simulink model "pp"  (R2021a)
settings: Solver=VariableStepAuto  StartTime=0.0  StopTime=10  RelTol=1e-3
values from neighbouring files (symbols this model uses):
  bound = 1e-6    (= 1e-06)    [parameter_setting.m]
  degree = 0.5    [parameter_setting.m]
  N = 2    [ICL_offline.m]
  rp = [-0.1 0 0.1]    [parameter_setting.m]
undefined symbols (not defined in the file or in its folder): DiscIntNeverNeededParam, Levenberg, Marquardt, sigbuilder_block, X, Y, Z
libraries: sm_lib x161, nesl_utility x35, robotmaniplib x2
(part 5 of 5)

== matlab function pp/Controller ==
  settings: updateMethod=DISCRETE  sampleTime=0.0001
  data: ref input; tau_1 output; tau_2 output; rp input; state input; wrench input; t input; aa output; b output; c output; dbg output; dbg1 output; dbg2 output; dbg3 output; dbg4 output
function [tau_1,tau_2,aa, b, c, dbg, dbg1, dbg2, dbg3, dbg4] = fcn(ref, rp, state, wrench, t)
%% gains
% robot number
N = 2;

% ICL gain
N_o = 10;
eason_integral = 4;
ICL_switcher = true;
k_cl_m = 2;
k_cl_rp = 1;
k_cl_I = 1;
k_cl_Ixx = 100; %100
k_cl_Iyy = 25; %25
k_cl_Izz = 15;
k_cl_ri = 10;
k_cl = [k_cl_m k_cl_rp*ones(1,3) k_cl_Ixx k_cl_I k_cl_I k_cl_Iyy k_cl_I k_cl_Izz k_cl_ri*ones(1,3*N)];
k_cl_gain = diag(k_cl);

% gamma o
g_m = 1;
g_rp = 1;
g_I = 1;
g_Ixx = 1;
g_Iyy = 1;
g_Izz = 1;
g_ri = 1;
gg = [g_m g_rp*ones(1,3) g_Ixx g_I g_I g_Iyy g_I g_Izz g_ri*ones(1,3*N)];
g_o = diag(gg);

% Kd matrix
Kdl = 1;
kdz = 20;
Kdr = 5;
Kdd = [Kdl*ones(1,2) kdz Kdr*ones(1,3)];
Kd = diag(Kdd);

% sliding parameter
lambda = 3;

% deadband in which to stop adaptation
deadband = 0.00;

%% function definition
function output = vee(matrix)
    output = [matrix(3, 2); matrix(1, 3); matrix(2, 1)];
end

function output = Pa(matrix)
    output = 0.5 * (matrix - matrix.');
end

function output = skew(v)
   output =  [    0 -v(3)   v(2)
               v(3)     0  -v(1)
              -v(2)  v(1)      0];
end

function output = L(v)
    output = [v(1)  v(2)  v(3)     0     0     0
                 0  v(1)     0  v(2)  v(3)     0
                 0     0  v(1)     0  v(2)  v(3)];
end
%% initialize
persistent v_last;
persistent w_last;
persistent index;
persistent mat_matrix;
persistent theta_o_hat;
persistent theta_o;
persistent Rd;
persistent xd;
persistent ICL_update;
persistent t_last;
persistent eason_ptr;

if isempty(index)
        % ground truth
        mass = 2;
        center_of_mass = rp;
        inertia_matrix = [0.0133333, 0, 0, 0.113333, 0, 0.113333];
        r1 = [-0.4 0 0] - rp;
        r2 = [0.4 0 0] - rp;
        r = [r1, r2];
        if N == 1
            theta_o = [mass mass*center_of_mass inertia_matrix r1].';
        else
            theta_o = [mass mass*center_of_mass inertia_matrix r].';
        end
        
        % initial guess
        theta_o_hat = zeros(10 + 3 * N, 1);
        theta_o_hat = theta_o;
        % mass
        theta_o_hat(1) = 0;
        % COG
        theta_o_hat(2) = 0;
        theta_o_hat(3) = 0;
        theta_o_hat(4) = 0;
        % Inertia
        theta_o_hat(5) = 0.0;
        theta_o_hat(6) = 0.0;
        theta_o_hat(7) = 0.0;
        theta_o_hat(8) = 0.0;
        theta_o_hat(9) = 0.0;
        theta_o_hat(10) = 0.0;
        % 1st grasp point
        theta_o_hat(11) = 0;
        theta_o_hat(12) = 0;
        theta_o_hat(13) = 0;
        % 2nd grasp point
        if N == 2
            theta_o_hat(14) = 0;
            theta_o_hat(15) = 0;
            theta_o_hat(16) = 0;
        end
        
        % without ICL first time
        ICL_update = false;

        Rd = [1  0  0;
              0  1  0;
              0  0  1];

        xd = [0.8750; 0.1092; 0.42] + rp.';
        index = 1;
        v_last = zeros(3, 1);
        w_last = zeros(3, eason_integral);
        mat_matrix = zeros(size(theta_o_hat, 1), N_o);
        t_last = 0;
        eason_ptr = 1; 
end

mat_sum = zeros(size(theta_o_hat, 1), 1);
debug_msg = zeros(6, 1);
dt = t - t_last;
G = [0; 0; -9.80665];

%% unpack ref
vd = [ref(1); ref(2); ref(3)];
ad = [ref(4); ref(5); ref(6)];
wd = [ref(7); ref(8); ref(9)];
ald = [ref(10); ref(11); ref(12)];

%% unpack state
quat = [state(1) state(2) state(3) state(4)];
R = quat2rotm(quat);
w = [state(5); state(6); state(7)];
x = [state(8); state(9); state(10)];
v = [state(11); state(12); state(13)];
a = [state(14); state(15); state(16)];

wrench_rotation = [         R, zeros(3,3);
                   zeros(3,3),          R];
wrench1_b = [wrench(1); wrench(2); wrench(3); wrench(4); wrench(5); wrench(6)];
wrench_1 = wrench_rotation * wrench1_b;
force_1 = [wrench_1(1); wrench_1(2); wrench_1(3)];
if N == 2
    wrench2_b = [wrench(7); wrench(8); wrench(9); wrench(10); wrench(11); wrench(12)];
    wrench_2 = wrench_rotation * wrench2_b;
    force_2 = [wrench_2(1); wrench_2(2); wrench_2(3)];
end

%% compute error signals
Re = Rd.' * R;
we = w - wd;

%% compute composite error s
sigma = we + lambda * Rd * vee(Pa(Re));
v_t = v - vd;
x_t = x - xd;
s = [v_t + lambda * x_t;
                  sigma];

%% regression matrix
alpha_r = ald - lambda * skew(wd) * Rd * vee(Pa(Re)) - lambda * Rd * vee(Pa(skew(Rd.' * we) * Re));
w_r = wd - lambda * Rd * vee(Pa(Re));
a_r = ad - lambda * v_t;
v_r = vd - lambda * x_t;

Y_l = [a_r, -skew(alpha_r) * R - skew(w) * skew(w_r) * R, zeros(3,6+3*N)];
if N == 1
    Y_r = [zeros(3,1), skew(a_r) * R + skew(w) * skew(v_r) * R - skew(w_r) * skew(v) * R, R * L(R.' * alpha_r) + skew(w) * R * L(R.' * w_r), skew(force_1)*R];
else
    Y_r = [zeros(3,1), skew(a_r) * R + skew(w) * skew(v_r) * R - skew(w_r) * skew(v) * R, R * L(R.' * alpha_r) + skew(w) * R * L(R.' * w_r), skew(force_1)*R, skew(force_2)*R];
end
Y_o = [Y_l;
       Y_r];
   
%% ICL
if ICL_update && ICL_switcher
    y_l = [(a - G) * eason_integral * dt, -skew(w - w_last(:,eason_ptr)) * R - (skew(w) * skew(w) * R) * eason_integral * dt, zeros(3,6 + 3 * N)];
    if N == 1
        y_r = [zeros(3,1), skew(a - G) * R * eason_integral * dt, R * L(R.' * (w - w_last(:,eason_ptr))) + (skew(w) * R * L(R.' * w)) * eason_integral * dt, skew(force_1) * R * eason_integral * dt];
    else
        y_r = [zeros(3,1), skew(a - G) * R * eason_integral * dt, R * L(R.' * (w - w_last(:,eason_ptr))) + (skew(w) * R * L(R.' * w)) * eason_integral * dt, skew(force_1) * R * eason_integral * dt, skew(force_2) * R * eason_integral * dt];
    end

    y_o_cl_integral = [y_l;
                       y_r];

    if index > N_o
        index = 1;
    end

    if N == 1
        true_tau_integral = wrench_1 * eason_integral * dt;
    else
        true_tau_integral = (wrench_1 + wrench_2) * eason_integral * dt;
    end
    
    y_o_cl_integral_a_hat = y_o_cl_integral * theta_o_hat;
    mat_now = y_o_cl_integral.' * (y_o_cl_integral_a_hat - true_tau_integral);
    
    debug_msg = y_o_cl_integral * theta_o - true_tau_integral;

    
    mat_matrix(:, index) = mat_now;

    mat_sum = sum(mat_matrix, 2);

    index = index + 1;

    v_last = v;
    w_last(:,eason_ptr) = w;
    if eason_ptr >= eason_integral
        eason_ptr = 1;
    else
        eason_ptr = eason_ptr + 1;
    end
end

t_last = t;

theta_o_hat_dot = zeros(10 + 3 * N, 1);
if ICL_update && ICL_switcher
    theta_o_hat_dot = -g_o * Y_o.' * s - k_cl_gain * g_o * mat_sum;
else
    theta_o_hat_dot = -g_o * Y_o.' * s;
end

% decide whether update or not
if norm(s) < deadband
    ICL_update = false;
else
    ICL_update = true;
end

%% desired signal calculate
Rd = expm(dt * skew(wd)) * Rd; % Matrix Exponential
xd = xd + vd * dt + 0.5 * ad * dt * dt;

%% update law
theta_o_hat = theta_o_hat + theta_o_hat_dot * dt;
theta_o_hat(5:10) = max(theta_o_hat(5:10), 0);

%% controller
tau = -Kd * s;
tau = min(max(tau, -20),40);

%% debug


%% output
tau_1 = tau + Y_o * theta_o_hat;
tau_2 = tau + Y_o * theta_o_hat;
aa = xd;
b = x;
c = theta_o_hat;
dbg = s;
dbg1 = wd;
dbg2 = expm(dt * skew(wd));
dbg3 = Rd;
dbg4 = R;
end

== matlab function pp/TH Magic/Arm 1 Magic/Transformation ==
  settings: updateMethod=DISCRETE  sampleTime=0.0005
  data: translation input; RPY input; T output
function T = fcn(translation, RPY)
    persistent R;
    persistent R_i;
    if isempty(R)
%         R = diag(ones(1,3));
         R = [1     0     0;
              0    -1     0;
              0     0    -1];
         R_i = R;
    end

R = rotx(RPY(1)) * roty(RPY(2)) * rotz(RPY(3)) * R; % *180/pi
T = [R translation;
     zeros(1,3)  1
    ];

== matlab function pp/TH Magic/Arm 2 Magic/Transformation ==
  settings: updateMethod=DISCRETE  sampleTime=0.0005
  data: translation input; RPY input; T output
function T = fcn(translation, RPY)
    persistent R;
    persistent R_i;
    if isempty(R)
%         R = diag(ones(1,3));
         R = [1     0     0;
              0    -1     0;
              0     0    -1];
         R_i = R;
    end

R = rotx(RPY(1)) * roty(RPY(2)) * rotz(RPY(3)) * R; % *180/pi
T = [R translation;
     zeros(1,3)  1
    ];
